simulink model "flightControlSystem"  (R2019a)
settings: Solver=ode3  StartTime=0  StopTime=TFinal  FixedStep=Ts  RelTol=1e-3  EnableMultiTasking=on
undefined symbols (not defined in the file): codertarget, Controller, DiscIntNeverNeededParam, Discrete, Estimator, g, init, Sensors, Time, Ts, Vehicle
libraries: simulink x37, sharedtransform x3, ctrlSharedLib x2, sharedutil x1, parrotlib x1
(part 1 of 2)
settings Model: ExtModeTrigDuration=80  Creator=The MathWorks, Inc.  LastModifiedBy=jeiso
settings SolverCC: AutoInsertRateTranBlk=on
settings DataIOCC: LimitDataPoints=on  SaveFormat=StructureWithTime  ReturnWorkspaceOutputs=off
settings OptimizationCC: BlockReduction=off  EnhancedBackFolding=on  PassReuseOutputArgsAs=Individual arguments  MaxStackSize=64  OptimizeBlockOrder=speed  DifferentSizesBufferReuse=on  OptimizationCustomize=off
settings DebuggingCC: AlgebraicLoopMsg=none  ParameterPrecisionLossMsg=none  ParameterTunabilityLossMsg=error  UnconnectedInputMsg=none  UnconnectedOutputMsg=none  UnconnectedLineMsg=none  BusObjectLabelMismatch=error  PregeneratedLibrarySubsystemCodeDiagnostic=none  SFUnexpectedBacktrackingDiag=warning  SFNoUnconditionalDefaultTransitionDiag=warning  SFExecutionAtInitializationDiag=none  ArithmeticOperatorsInVariantConditions=warning
settings HardwareCC: ProdBitPerPointer=32  ProdBitPerSizeT=32  ProdBitPerPtrDiffT=32  ProdLargestAtomicInteger=Long  ProdWordSize=32  ProdHWDeviceType=ARM Compatible->ARM 9  UseEmbeddedCoderFeatures=off  UseSimulinkCoderFeatures=off
settings ModelReferenceCC: ModelReferenceNumInstancesAllowed=Single  PropagateSignalLabelsOutOfModel=off
settings SFSimCC: SimUseLocalCustomCode=off  MATLABDynamicMemAlloc=off
settings RTWCC: SystemTargetFile=ert.tlc  HardwareBoard=PARROT Mambo  TLCOptions=-aInlineSetEventsForThisBaseRateFcn=TLC_FALSE -aSuppressMultiTaskScheduler=TLC_FALSE -aRateBasedStepFcn=1  TemplateMakefile=ert_default_tmf  RTWUseLocalCustomCode=off  Toolchain=Sourcery G++ Lite GNU Toolchain for Drones  IncludeHyperlinkInReport=on
settings CodeAppCC: ForceParamTrailComments=on  IgnoreCustomStorageClasses=off  MaxIdLength=63  OperatorAnnotations=on  SimulinkDataObjDesc=on  SFDataObjDesc=on  InsertBlockDesc=on
settings ERTTargetCC: MatFileLogging=on  SupportNonInlinedSFcns=on
settings ConfigComp: CovMetricSettings=dw  CovHtmlReporting=on  CovSaveCumulativeToWorkspaceVar=on  CovSaveSingleToWorkspaceVar=on  CovExternalEMLEnable=off  CovSFcnEnable=off

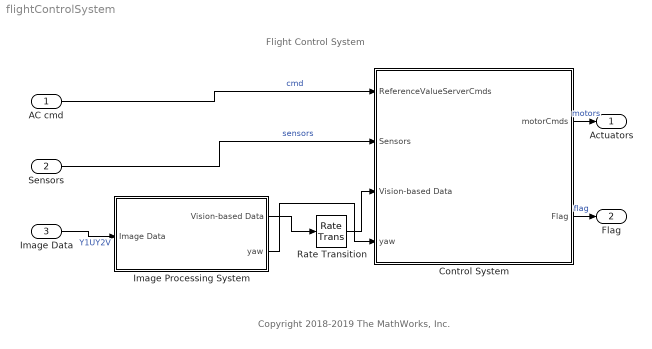
== system flightControlSystem ==
  note: Copyright 2018-2019 The MathWorks, Inc.
  note: Flight Control System
  AC cmd : Inport  OutDataTypeStr=Bus: CommandBus  BusOutputAsStruct=on
  Sensors : Inport  Port=2  OutDataTypeStr=Bus: SensorsBus  BusOutputAsStruct=on
  Image Data : Inport  Tag=IP_IN  InitFcn=codertarget.parrot.internal.inportCallback(gcb);  Port=3  OutDataTypeStr=uint8  PortDimensions=[4 9600]  BusOutputAsStruct=on
  Control System : Subsystem  InitFcn=codertarget.parrot.internal.fcsSubsystemCallback(gcb);  TreatAsAtomicUnit=on  SystemSampleTime=Ts
  Image Processing System : Subsystem  Tag=IP_SUB  InitFcn=codertarget.parrot.internal.ipSubsystemCallback(gcb);  TreatAsAtomicUnit=on  SystemSampleTime=40*Ts  RTWFcnName=ImageFunction
      settings: RTWSystemCode=Inline  RTWFcnNameOpts=User specified
  Rate Transition : RateTransition  Deterministic=off
  Actuators : Outport  OutDataTypeStr=single  PortDimensions=4
  Flag : Outport  Port=2  OutDataTypeStr=uint8  PortDimensions=1
  wires:
  AC cmd/1 -> Control System/1(ReferenceValueServerCmds)  "cmd"
  Control System/1(motorCmds) -> Actuators/1  "motors"
  Sensors/1 -> Control System/2(Sensors)  "sensors"
  Control System/2(Flag) -> Flag/1  "flag"
  Image Data/1 -> Image Processing System/1(Image Data)  "Y1UY2V"
  Image Processing System/1(Vision-based Data) -> Rate Transition/1
  Rate Transition/1 -> Control System/3(Vision-based Data)
  Image Processing System/2("yaw ") -> Control System/4(" yaw")

== system flightControlSystem/Control System ==
  note: Position or Orientation Control
  note: Use this subsystem to change the path of the
      | Minidrone depending on the input Vision-based
      | Data
  note: Derived from the work by Sertac
      | Karaman and Fabian Riether
  ReferenceValueServerCmds : Inport  OutDataTypeStr=Bus: CommandBus
  Sensors : Inport  Port=2  OutDataTypeStr=Bus: SensorsBus  BusOutputAsStruct=on
  Vision-based Data : Inport  Port=3
  " yaw" : Inport  Port=4
  Bus Selector1 : BusSelector  OutputSignals=opticalFlow_data
  Bus Selector4 : BusSelector  OutputSignals=VisionSensors,SensorCalibration
  Control Mode Update : BusAssignment  AssignedSignals=controlModePosVSOrient
  Controller : Subsystem
  Crash Predictor Flags : Subsystem
  Path Planning : Subsystem
  State Estimator : Subsystem
  To Workspace : ToWorkspace  VariableName=estimatedStates  SaveFormat=Structure With Time  SampleTime=-1
  controlModePosVsOrient : Constant  OutDataTypeStr=boolean
  motorCmds : Outport
  Flag : Outport  Port=2
  wires:
  ReferenceValueServerCmds/1 -> Control Mode Update/1
  Bus Selector1/1 -> State Estimator/3(opticalFlow_datin)  "<opticalFlow_data>"
  Bus Selector4/2 -> State Estimator/4(sensorCalibration_datin)  "<SensorCalibration>"
  Path Planning/1(UpdatedReferenceCmds) -> Controller/1(ReferenceValueServerBus)
  Bus Selector4/1 -> Bus Selector1/1  "<VisionSensors>"
  Vision-based Data/1 -> Path Planning/4(rojo)
  Crash Predictor Flags/1(Flag) -> Flag/1
  Control Mode Update/1 -> Path Planning/1(ReferenceValueServerCmds)
  controlModePosVsOrient/1 -> State Estimator/1(controlModePosVSOrient_flagin), Control Mode Update/2
  Controller/1(motors_refout) -> motorCmds/1
  Sensors/1 -> State Estimator/2(sensor_data_in), Crash Predictor Flags/3(Sensors), Bus Selector4/1
  State Estimator/1(states_estim) -> Path Planning/2(EstimatedVal), Controller/2(states_estim), Crash Predictor Flags/1(states_estim), To Workspace/1
  State Estimator/2(Alt_prs) -> Crash Predictor Flags/2(Alt_prs)
  " yaw"/1 -> Path Planning/3(grados)
  Path Planning/2("yaw ") -> Controller/3("yaw ")

== system flightControlSystem/Image Processing System ==
  note: Find the dominance of blue in the image
  note: Find the B-(R/2)-(G/2) image
  note: Obtain the RGB image from camera
  Image Data : Inport
  Add : Sum  Inputs=--+
  Constant : Constant  Value=2
  Delay : Delay  DelayLength=1
  Deteccion de giros : MATLAB Function  TreatAsAtomicUnit=on
  Display : Display
  Display1 : Display
  Divide1 : Product  Inputs=/*
  Divide2 : Product  Inputs=*/
  PARROT Image Conversion : parrotlib/PARROT Image Conversion  ImageFormat=RGB  R=on  Y=on  G=on  U=on  B=on  V=on
      settings: SourceProductName=Simulink Support Package for PARROT Minidrones
  RGB Image : VideoViewer  FigPos=[565 571 418 304]
  RGB Image1 : VideoViewer  FigPos=[896 489 418 304]
  Sum of white pixels : Sum  Inputs=+  OutDataTypeStr=uint16
  Threshold for each pixel : simulink/Logic and Bit Operations/Compare To Constant  relop=>  const=50  OutDataTypeStr=boolean
  Threshold for total white pixels : simulink/Logic and Bit Operations/Compare To Constant  relop=>  const=1400  OutDataTypeStr=boolean
  To Workspace : ToWorkspace  VariableName=simout  SaveFormat=Timeseries  SampleTime=-1
  Vision-based Data : Outport
  "yaw " : Outport  Port=2
  wires:
  Image Data/1 -> PARROT Image Conversion/1
  Threshold for total white pixels/1 -> Vision-based Data/1
  Add/1 -> Threshold for each pixel/1
  Sum of white pixels/1 -> Threshold for total white pixels/1
  Divide2/1 -> Add/1
  PARROT Image Conversion/3 -> Divide2/1
  PARROT Image Conversion/1 -> Add/3
  PARROT Image Conversion/2 -> Divide1/2
  Divide1/1 -> Add/2
  Constant/1 -> Divide1/1, Divide2/2
  Deteccion de giros/2(grados) -> Delay/1, "yaw "/1
  Deteccion de giros/4(imagen) -> RGB Image1/1
  Threshold for each pixel/1 -> Deteccion de giros/1(img), RGB Image/1, Sum of white pixels/1
  Deteccion de giros/3(lado) -> Display1/1
  Delay/1 -> Deteccion de giros/2(grado)
  Deteccion de giros/1(ade) -> To Workspace/1, Display/1

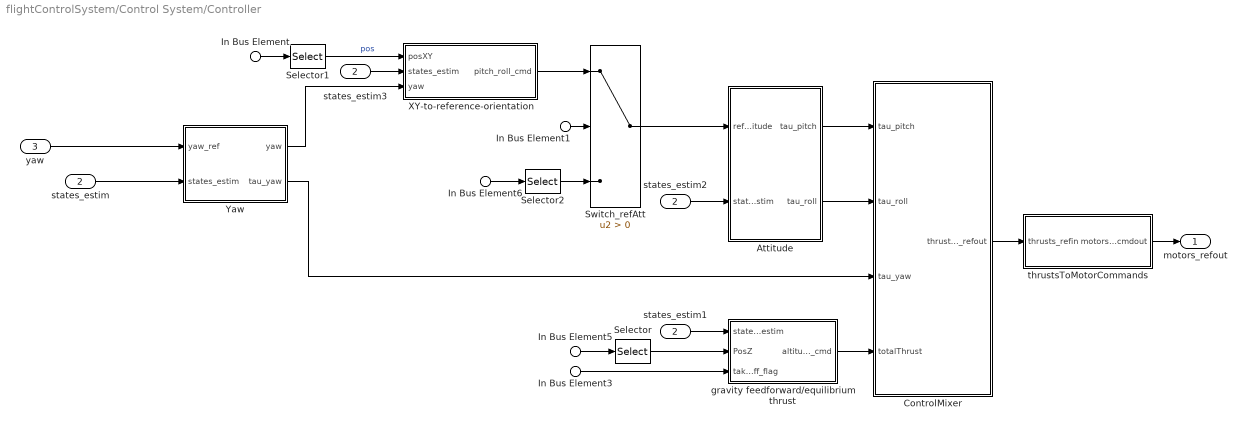
== system flightControlSystem/Control System/Controller ==
  In Bus Element1 : Inport  PortName=ReferenceValueServerBus  Element=controlModePosVSOrient
  In Bus Element : Inport  PortName=ReferenceValueServerBus  Element=pos_ref
  In Bus Element5 : Inport  PortName=ReferenceValueServerBus  Element=pos_ref
  In Bus Element6 : Inport  PortName=ReferenceValueServerBus  Element=orient_ref
  In Bus Element3 : Inport  PortName=ReferenceValueServerBus  Element=takeoff_flag
  states_estim : Inport  Port=2
  "yaw " : Inport  Port=3
  Attitude : Subsystem
  ControlMixer : Subsystem
  Selector : Selector  InputPortWidth=3  IndexOptions=Index vector (dialog)  Indices=3  OutputSizes=1
  Selector1 : Selector  InputPortWidth=3  IndexOptions=Index vector (dialog)  Indices=[1 2]  OutputSizes=1
  Selector2 : Selector  InputPortWidth=3  IndexOptions=Index vector (dialog)  Indices=[2 3]  OutputSizes=1
  Switch_refAtt : Switch  Criteria=u2 > Threshold
  XY-to-reference-orientation : Subsystem
  Yaw : Subsystem
  gravity feedforward/equilibrium thrust : Subsystem
  states_estim1 : InportShadow  Port=2
  states_estim2 : InportShadow  Port=2
  states_estim3 : InportShadow  Port=2
  thrustsToMotorCommands : Subsystem
  motors_refout : Outport
  wires:
  thrustsToMotorCommands/1(motors_cmdout) -> motors_refout/1
  In Bus Element5/1 -> Selector/1
  Attitude/2(tau_roll) -> ControlMixer/2(tau_roll)
  states_estim3/1 -> XY-to-reference-orientation/2(states_estim)
  In Bus Element6/1 -> Selector2/1
  "yaw "/1 -> Yaw/1(yaw_ref)
  In Bus Element/1 -> Selector1/1
  ControlMixer/1(thrusts_refout) -> thrustsToMotorCommands/1(thrusts_refin)
  Selector2/1 -> Switch_refAtt/3
  Attitude/1(tau_pitch) -> ControlMixer/1(tau_pitch)
  gravity feedforward/equilibrium thrust/1(altitude_cmd) -> ControlMixer/4(totalThrust)
  Selector1/1 -> XY-to-reference-orientation/1(posXY)  "pos"
  states_estim1/1 -> gravity feedforward/equilibrium thrust/1(states_estim)
  Selector/1 -> gravity feedforward/equilibrium thrust/2(PosZ)
  Yaw/1(yaw) -> XY-to-reference-orientation/3(yaw)
  In Bus Element3/1 -> gravity feedforward/equilibrium thrust/3(takeoff_flag)
  states_estim/1 -> Yaw/2(states_estim)
  XY-to-reference-orientation/1(pitch_roll_cmd) -> Switch_refAtt/1
  Yaw/2(tau_yaw) -> ControlMixer/3(tau_yaw)
  In Bus Element1/1 -> Switch_refAtt/2
  Switch_refAtt/1 -> Attitude/1(refAttitude)
  states_estim2/1 -> Attitude/2(states_estim)

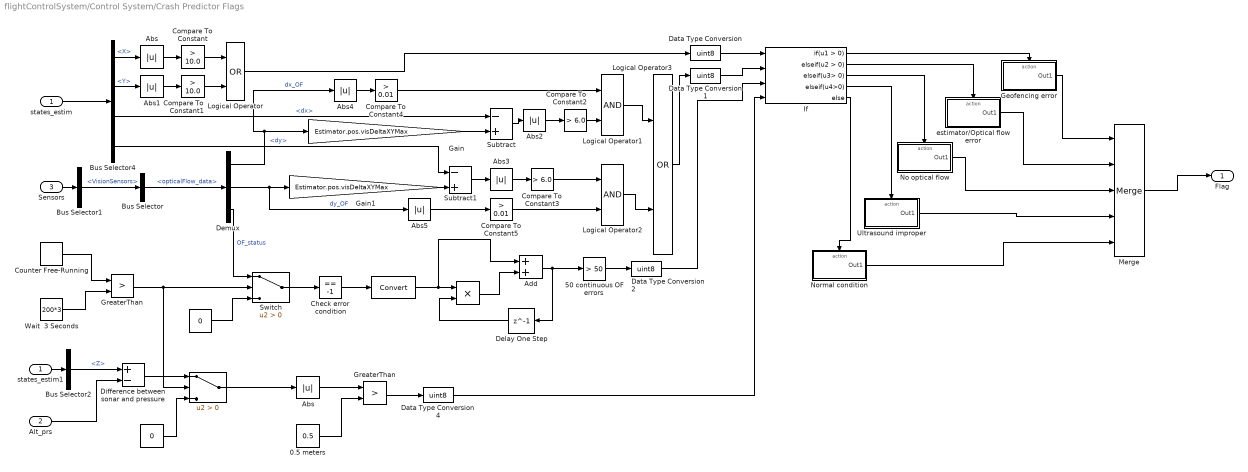
== system flightControlSystem/Control System/Crash Predictor Flags ==
  states_estim : Inport
  Alt_prs : Inport  Port=2
  Sensors : Inport  Port=3
  " " : Constant  Value=0
  "  " : Product  Inputs=**
  "   " : DataTypeConversion
  "    " : Constant  Value=0  OutDataTypeStr=single
  "         " : Switch  Criteria=u2 > Threshold
  0.5 meters : Constant  Value=0.5
  "50 continuous OF errors " : simulink/Logic and Bit Operations/Compare To Constant  relop=>  const=50  OutDataTypeStr=boolean
  Abs{,1..5} (6 alike) : Abs
  "Abs  " : Abs
  Add : Sum
  Bus Selector : BusSelector  OutputSignals=opticalFlow_data
  Bus Selector1 : BusSelector  OutputSignals=VisionSensors
  Bus Selector2 : BusSelector  OutputSignals=Z
  Bus Selector4 : BusSelector  OutputSignals=X,Y,dx,dy
  Check error condition : simulink/Logic and Bit Operations/Compare To Constant  relop===  const=-1  OutDataTypeStr=boolean
  Compare To Constant : simulink/Logic and Bit Operations/Compare To Constant  relop=>  const=10.0  OutDataTypeStr=boolean
  Compare To Constant1 : simulink/Logic and Bit Operations/Compare To Constant  relop=>  const=10.0  OutDataTypeStr=boolean
  Compare To Constant2 : simulink/Logic and Bit Operations/Compare To Constant  relop=>  const=6.0  OutDataTypeStr=boolean
  Compare To Constant3 : simulink/Logic and Bit Operations/Compare To Constant  relop=>  const=6.0  OutDataTypeStr=boolean
  Compare To Constant4 : simulink/Logic and Bit Operations/Compare To Constant  relop=>  const=0.01  OutDataTypeStr=boolean
  Compare To Constant5 : simulink/Logic and Bit Operations/Compare To Constant  relop=>  const=0.01  OutDataTypeStr=boolean
  Counter Free-Running : simulink/Sources/Counter Free-Running  NumBits=32  tsamp=-1
  Data Type Conversion{,1..2,4} (4 alike) : DataTypeConversion  OutDataTypeStr=uint8  RndMeth=Nearest
  Delay One Step : Delay  DelayLength=1
  Demux : Demux  Outputs=3
  Difference between sonar and pressure : Sum  Inputs=+-
  Gain : Gain  Gain=Estimator.pos.visDeltaXYMax
  Gain1 : Gain  Gain=Estimator.pos.visDeltaXYMax
  Geofencing error : Subsystem  TreatAsAtomicUnit=on
  GreaterThan : RelationalOperator  Operator=>  OutDataTypeStr=boolean  RndMeth=Simplest
  "GreaterThan  " : RelationalOperator  Operator=>  OutDataTypeStr=boolean  RndMeth=Simplest
  If : If  NumInputs=4  ElseIfExpressions=u2 > 0, u3> 0,u4>0
  Logical Operator : Logic  Operator=OR  AllPortsSameDT=off
  Logical Operator1 : Logic  AllPortsSameDT=off  OutDataTypeStr=boolean
  Logical Operator2 : Logic  AllPortsSameDT=off  OutDataTypeStr=boolean
  Logical Operator3 : Logic  Operator=OR  AllPortsSameDT=off
  Merge : Merge  Inputs=5  InitialOutput=0
  "No optical flow " : Subsystem  TreatAsAtomicUnit=on
  Normal condition : Subsystem  TreatAsAtomicUnit=on
  Subtract : Sum  Inputs=-+
  Subtract1 : Sum  Inputs=-+
  Switch : Switch  Criteria=u2 > Threshold
  Ultrasound improper : Subsystem  TreatAsAtomicUnit=on
  Wait  3 Seconds : Constant  Value=200*3
  estimator/Optical flow error : Subsystem  TreatAsAtomicUnit=on
  states_estim1 : InportShadow
  Flag : Outport
  wires:
  Bus Selector4/1 -> Abs/1  "<X>"
  states_estim/1 -> Bus Selector4/1
  Bus Selector4/2 -> Abs1/1  "<Y>"
  Compare To Constant/1 -> Logical Operator/1
  Compare To Constant1/1 -> Logical Operator/2
  Abs/1 -> Compare To Constant/1
  Abs1/1 -> Compare To Constant1/1
  Logical Operator/1 -> Data Type Conversion/1
  Bus Selector/1 -> Demux/1  "<opticalFlow_data>"
  Demux/1 -> Abs4/1, Gain/1  "dx_OF"
  Demux/2 -> Gain1/1, Abs5/1  "dy_OF"
  Bus Selector4/3 -> Subtract/1  "<dx>"
  Subtract/1 -> Abs2/1
  Subtract1/1 -> Abs3/1
  Abs2/1 -> Compare To Constant2/1
  Abs3/1 -> Compare To Constant3/1
  Compare To Constant5/1 -> Logical Operator2/2
  Abs4/1 -> Compare To Constant4/1
  Abs5/1 -> Compare To Constant5/1
  Compare To Constant3/1 -> Logical Operator2/1
  Logical Operator1/1 -> Logical Operator3/1
  Logical Operator2/1 -> Logical Operator3/2
  Logical Operator3/1 -> Data Type Conversion1/1
  Gain/1 -> Subtract/2
  Bus Selector4/4 -> Subtract1/1  "<dy>"
  Gain1/1 -> Subtract1/2
  Compare To Constant4/1 -> Logical Operator1/1
  Compare To Constant2/1 -> Logical Operator1/2
  Sensors/1 -> Bus Selector1/1
  Bus Selector1/1 -> Bus Selector/1  "<VisionSensors>"
  Merge/1 -> Flag/1
  If/1 -> Geofencing error/Action
  If/2 -> estimator/Optical flow error/Action
  If/5 -> Normal condition/Action
  Geofencing error/1(Out1) -> Merge/1
  estimator/Optical flow error/1(Out1) -> Merge/2
  Normal condition/1(Out1) -> Merge/5
  Data Type Conversion/1 -> If/1
  Data Type Conversion1/1 -> If/2
  Check error condition/1 -> "   "/1
  Demux/3 -> Switch/1  "OF_status"
  Delay One Step/1 -> "  "/2
  Add/1 -> Delay One Step/1, "50 continuous OF errors "/1
  "  "/1 -> Add/2
  "50 continuous OF errors "/1 -> Data Type Conversion2/1
  Data Type Conversion2/1 -> If/3
  "No optical flow "/1(Out1) -> Merge/3
  If/3 -> "No optical flow "/Action
  "   "/1 -> Add/1, "  "/1
  Counter Free-Running/1 -> GreaterThan/1
  Wait  3 Seconds/1 -> GreaterThan/2
  Switch/1 -> Check error condition/1
  " "/1 -> Switch/3
  "    "/1 -> "         "/3
  Difference between sonar and pressure/1 -> "         "/1
  Bus Selector2/1 -> Difference between sonar and pressure/1  "<Z>"
  GreaterThan/1 -> Switch/2, "         "/2
  "         "/1 -> "Abs  "/1
  "Abs  "/1 -> "GreaterThan  "/1
  0.5 meters/1 -> "GreaterThan  "/2
  Alt_prs/1 -> Difference between sonar and pressure/2
  "GreaterThan  "/1 -> Data Type Conversion4/1
  states_estim1/1 -> Bus Selector2/1
  Data Type Conversion4/1 -> If/4
  Ultrasound improper/1(Out1) -> Merge/4
  If/4 -> Ultrasound improper/Action

== system flightControlSystem/Control System/Path Planning ==
  note: Estimated values from the
      | State Estimator
  ReferenceValueServerCmds : Inport
  EstimatedVal : Inport  Port=2
  grados : Inport  Port=3
  rojo : Inport  Port=4
  Bus Selector1 : BusSelector  OutputSignals=X,Y,Z,yaw,pitch,roll
  Bus Assignment : BusAssignment  AssignedSignals=pos_ref
  Chart : Stateflow chart  BlockKeywords=__PRM__SERIALIZED__DATA__:Stateflow Chart,Stateflow Diagram  TreatAsAtomicUnit=on
  Mux : Mux  Inputs=3
  Terminator3 : Terminator
  Terminator5 : Terminator
  Terminator6 : Terminator
  UpdatedReferenceCmds : Outport
  "yaw " : Outport  Port=2
  wires:
  Bus Assignment/1 -> UpdatedReferenceCmds/1
  ReferenceValueServerCmds/1 -> Bus Assignment/1
  EstimatedVal/1 -> Bus Selector1/1
  Bus Selector1/1 -> Chart/1(xest)  "<X>"
  Bus Selector1/2 -> Chart/2(yest)  "<Y>"
  Bus Selector1/3 -> Terminator3/1  "<Z>"
  Bus Selector1/4 -> Chart/5(yawest)  "<yaw>"
  Bus Selector1/5 -> Terminator5/1  "<pitch>"
  Bus Selector1/6 -> Terminator6/1  "<roll>"
  Mux/1 -> Bus Assignment/2
  grados/1 -> Chart/4(grados)
  Chart/4(yaw) -> "yaw "/1
  Chart/1(x) -> Mux/1
  Chart/2(y) -> Mux/2
  Chart/3(z) -> Mux/3
  rojo/1 -> Chart/3(rojo)

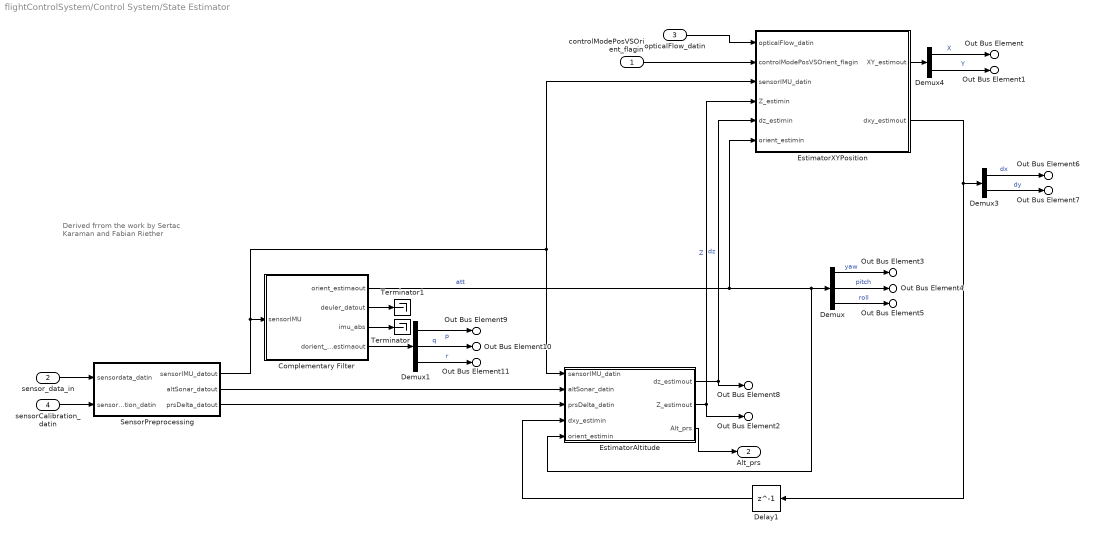
== system flightControlSystem/Control System/State Estimator ==
  note: Derived frrom the work by Sertac
      | Karaman and Fabian Riether
  controlModePosVSOrient_flagin : Inport  OutDataTypeStr=boolean
  sensor_data_in : Inport  Port=2
  opticalFlow_datin : Inport  Port=3
  sensorCalibration_datin : Inport  Port=4
  Complementary Filter : Subsystem
  Delay1 : Delay  DelayLength=1  InitialCondition=0
  Demux : Demux  Outputs=3
  Demux1 : Demux  Outputs=3
  Demux3 : Demux  Outputs=2
  Demux4 : Demux  Outputs=2
  EstimatorAltitude : Subsystem
  EstimatorXYPosition : Subsystem
  SensorPreprocessing : Subsystem
  Terminator : Terminator
  Terminator1 : Terminator
  Out Bus Element : Outport  PortName=states_estim  Element=X
  Out Bus Element1 : Outport  PortName=states_estim  Element=Y
  Out Bus Element2 : Outport  PortName=states_estim  Element=Z
  Out Bus Element3 : Outport  PortName=states_estim  Element=yaw
  Out Bus Element4 : Outport  PortName=states_estim  Element=pitch
  Out Bus Element5 : Outport  PortName=states_estim  Element=roll
  Out Bus Element6 : Outport  PortName=states_estim  Element=dx
  Out Bus Element7 : Outport  PortName=states_estim  Element=dy
  Out Bus Element8 : Outport  PortName=states_estim  Element=dz
  Out Bus Element9 : Outport  PortName=states_estim  Element=p
  Out Bus Element10 : Outport  PortName=states_estim  Element=q
  Out Bus Element11 : Outport  PortName=states_estim  Element=r
  Alt_prs : Outport  Port=2
  wires:
  EstimatorXYPosition/2(dxy_estimout) -> Delay1/1, Demux3/1
  Demux1/3 -> Out Bus Element11/1  "r"
  Demux/3 -> Out Bus Element5/1  "roll"
  Demux4/2 -> Out Bus Element1/1  "Y"
  EstimatorXYPosition/1(XY_estimout) -> Demux4/1
  Complementary Filter/2(deuler_datout) -> Terminator1/1
  Complementary Filter/4(dorient_estimaout) -> Demux1/1
  sensor_data_in/1 -> SensorPreprocessing/1(sensordata_datin)
  opticalFlow_datin/1 -> EstimatorXYPosition/1(opticalFlow_datin)
  Demux4/1 -> Out Bus Element/1  "X"
  SensorPreprocessing/1(sensorIMU_datout) -> EstimatorAltitude/1(sensorIMU_datin), EstimatorXYPosition/3(sensorIMU_datin), Complementary Filter/1(sensorIMU)
  SensorPreprocessing/3(prsDelta_datout) -> EstimatorAltitude/3(prsDelta_datin)
  Demux3/2 -> Out Bus Element7/1  "dy"
  SensorPreprocessing/2(altSonar_datout) -> EstimatorAltitude/2(altSonar_datin)
  EstimatorAltitude/1(dz_estimout) -> EstimatorXYPosition/5(dz_estimin), Out Bus Element8/1  "dz"
  EstimatorAltitude/2(Z_estimout) -> Out Bus Element2/1, EstimatorXYPosition/4(Z_estimin)  "Z"
  Demux1/1 -> Out Bus Element9/1  "p"
  Demux3/1 -> Out Bus Element6/1  "dx"
  Complementary Filter/3(imu_abs) -> Terminator/1
  Demux/2 -> Out Bus Element4/1  "pitch"
  controlModePosVSOrient_flagin/1 -> EstimatorXYPosition/2(controlModePosVSOrient_flagin)
  Complementary Filter/1(orient_estimaout) -> EstimatorAltitude/5(orient_estimin), Demux/1, EstimatorXYPosition/6(orient_estimin)  "att"
  Demux/1 -> Out Bus Element3/1  "yaw"
  Delay1/1 -> EstimatorAltitude/4(dxy_estimin)
  Demux1/2 -> Out Bus Element10/1  "q"
  sensorCalibration_datin/1 -> SensorPreprocessing/2(sensorCalibration_datin)
  EstimatorAltitude/3(Alt_prs) -> Alt_prs/1

== system flightControlSystem/Control System/Controller/Attitude ==
  note: ATTITUDE
  refAttitude : Inport
  states_estim : Inport  Port=2
  Add : Sum  Inputs=+-
  Bus Selector3 : BusSelector  OutputSignals=pitch,roll
  Bus Selector4 : BusSelector  OutputSignals=q,p
  D_pr : Gain  Gain=[0.002;0.003]
  Delay : Delay  DelayLength=1  InitialCondition=0
  Demux : Demux  Outputs=2
  Discrete-Time Integrator : DiscreteIntegrator  SampleTime=Ts  LimitOutput=on  UpperSaturationLimit=2  LowerSaturationLimit=-2  ICPrevOutput=DiscIntNeverNeededParam  ICPrevScaledInput=DiscIntNeverNeededParam
  I_pr : Gain  Gain=0.01
  Mux : Mux  Inputs=2
  Mux1 : Mux  Inputs=2
  P_pr : Gain  Gain=[0.013;0.011]
  Sum16 : Sum  Inputs=++-  AccumDataTypeStr=single  OutDataTypeStr=single  SaturateOnIntegerOverflow=on
  Sum19 : Sum  Inputs=+-|
  antiWU_Gain : Gain  Gain=0.001
  tau_pitch : Outport
  tau_roll : Outport  Port=2
  wires:
  Sum16/1 -> Demux/1  "P_pr"
  antiWU_Gain/1 -> Add/2
  Add/1 -> Discrete-Time Integrator/1
  Bus Selector3/1 -> Mux/1  "<pitch>"
  Bus Selector4/1 -> Mux1/1  "<q>"
  P_pr/1 -> Sum16/1
  I_pr/1 -> Sum16/2
  Sum19/1 -> Add/1, P_pr/1  "pitch/roll error"
  Discrete-Time Integrator/1 -> Delay/1, I_pr/1
  Delay/1 -> antiWU_Gain/1
  Demux/1 -> tau_pitch/1  "tau_pitch"
  Demux/2 -> tau_roll/1
  D_pr/1 -> Sum16/3
  states_estim/1 -> Bus Selector3/1, Bus Selector4/1
  refAttitude/1 -> Sum19/1
  Mux/1 -> Sum19/2
  Bus Selector3/2 -> Mux/2  "<roll>"
  Mux1/1 -> D_pr/1
  Bus Selector4/2 -> Mux1/2  "<p>"

== system flightControlSystem/Control System/Controller/ControlMixer ==
  tau_pitch : Inport
  tau_roll : Inport  Port=2
  tau_yaw : Inport  Port=3
  totalThrust : Inport  Port=4
  Mux2 : Mux
  Product : Product  Multiplication=Matrix(*)  RndMeth=Zero
  TorqueTotalThrustToThrustPerMotor : Constant  Value=Controller.Q2Ts  OutDataTypeStr=single
  thrusts_refout : Outport
  wires:
  Product/1 -> thrusts_refout/1
  tau_roll/1 -> Mux2/4
  tau_pitch/1 -> Mux2/3
  tau_yaw/1 -> Mux2/2
  totalThrust/1 -> Mux2/1
  TorqueTotalThrustToThrustPerMotor/1 -> Product/1
  Mux2/1 -> Product/2

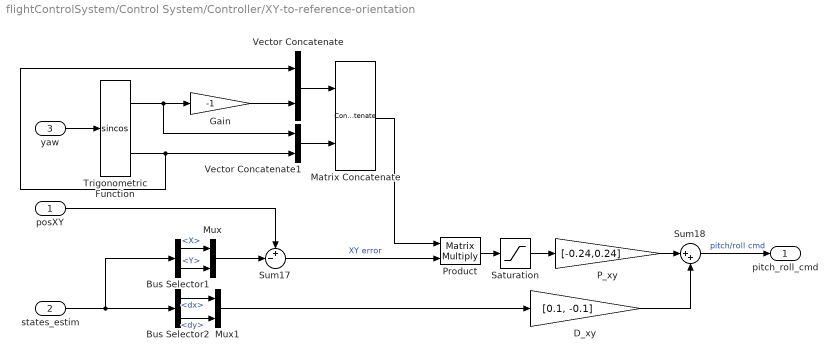
== system flightControlSystem/Control System/Controller/XY-to-reference-orientation ==
  posXY : Inport
  states_estim : Inport  Port=2
  yaw : Inport  Port=3
  Bus Selector1 : BusSelector  OutputSignals=X,Y
  Bus Selector2 : BusSelector  OutputSignals=dx,dy
  D_xy : Gain  Gain=[0.1, -0.1]  ParamDataTypeStr=single  OutDataTypeStr=single  SaturateOnIntegerOverflow=on
  Gain : Gain  Gain=-1
  Matrix Concatenate : Concatenate  Mode=Multidimensional array  ConcatenateDimension=2
  Mux : Mux  Inputs=2
  Mux1 : Mux  Inputs=2
  P_xy : Gain  Gain=[-0.24,0.24]  ParamDataTypeStr=single  OutDataTypeStr=single  SaturateOnIntegerOverflow=on
  Product : Product  Multiplication=Matrix(*)  OutDataTypeStr=single  RndMeth=Zero
  Saturation : Saturate  UpperLimit=3  LowerLimit=-3  OutDataTypeStr=single
  Sum17 : Sum  Inputs=+-|  AccumDataTypeStr=single
  Sum18 : Sum  Inputs=|++  AccumDataTypeStr=single  OutDataTypeStr=single  SaturateOnIntegerOverflow=on
  Trigonometric Function : Trigonometry  Operator=sincos
  Vector Concatenate : Concatenate
  Vector Concatenate1 : Concatenate
  pitch_roll_cmd : Outport
  wires:
  yaw/1 -> Trigonometric Function/1
  Saturation/1 -> P_xy/1
  P_xy/1 -> Sum18/1
  Sum17/1 -> Product/2  "XY error"
  posXY/1 -> Sum17/1
  Bus Selector2/1 -> Mux1/1  "<dx>"
  states_estim/1 -> Bus Selector1/1, Bus Selector2/1
  Sum18/1 -> pitch_roll_cmd/1  "pitch/roll cmd"
  D_xy/1 -> Sum18/2
  Bus Selector1/1 -> Mux/1  "<X>"
  Product/1 -> Saturation/1
  Trigonometric Function/1 -> Gain/1, Vector Concatenate1/1
  Trigonometric Function/2 -> Vector Concatenate1/2, Vector Concatenate/1
  Gain/1 -> Vector Concatenate/2
  Vector Concatenate/1 -> Matrix Concatenate/1
  Vector Concatenate1/1 -> Matrix Concatenate/2
  Matrix Concatenate/1 -> Product/1
  Bus Selector1/2 -> Mux/2  "<Y>"
  Mux/1 -> Sum17/2
  Mux1/1 -> D_xy/1
  Bus Selector2/2 -> Mux1/2  "<dy>"

== system flightControlSystem/Control System/Controller/Yaw ==
  yaw_ref : Inport
  states_estim : Inport  Port=2
  Bus Selector5 : BusSelector  OutputSignals=yaw,r
  D_yaw : Gain  Gain=0.3*0.004
  P_yaw : Gain  Gain=0.004  ParamDataTypeStr=single  OutDataTypeStr=single
  Sum1 : Sum  Inputs=+-|  AccumDataTypeStr=single  OutDataTypeStr=single  SaturateOnIntegerOverflow=on
  Sum2 : Sum  Inputs=|+-
  yaw : Outport
  tau_yaw : Outport  Port=2
  wires:
  D_yaw/1 -> Sum2/2
  P_yaw/1 -> Sum2/1
  Bus Selector5/2 -> D_yaw/1  "<r>"
  Sum1/1 -> P_yaw/1
  states_estim/1 -> Bus Selector5/1
  Sum2/1 -> tau_yaw/1
  Bus Selector5/1 -> yaw/1, Sum1/2  "<yaw>"
  yaw_ref/1 -> Sum1/1

== system flightControlSystem/Control System/Controller/gravity feedforward//equilibrium thrust ==
  note: ALTITUDE
  states_estim : Inport
  PosZ : Inport  Port=2
  takeoff_flag : Inport  Port=3
  Bus Selector1 : BusSelector  OutputSignals=Z,dz
  Compare To Constant : simulink/Logic and Bit Operations/Compare To Constant  relop=<  const=100  OutDataTypeStr=boolean
  Counter Free-Running : simulink/Sources/Counter Free-Running  NumBits=32  tsamp=-1
  D_z1 : Gain  Gain=0.5  ParamDataTypeStr=single  OutDataTypeStr=single  SaturateOnIntegerOverflow=on
  Discrete-Time Integrator : DiscreteIntegrator  ExternalReset=falling  SampleTime=Ts  LimitOutput=on  UpperSaturationLimit=2  LowerSaturationLimit=-2  ICPrevOutput=DiscIntNeverNeededParam  ICPrevScaledInput=DiscIntNeverNeededParam
  I_pr : Gain  Gain=0.24
  P_z1 : Gain  Gain=0.8  ParamDataTypeStr=single  OutDataTypeStr=single  SaturateOnIntegerOverflow=on
  SaturationThrust1 : Saturate  UpperLimit=4*Controller.totalThrustMaxRelative*Controller.motorsThrustPerMotorMax  LowerLimit=-4*Controller.totalThrustMaxRelative*Controller.motorsThrustPerMotorMax  OutDataTypeStr=single
  Sum1 : Sum  Inputs=++-  AccumDataTypeStr=single  OutDataTypeStr=single  SaturateOnIntegerOverflow=on
  Sum2 : Sum  Inputs=+-|  AccumDataTypeStr=single  OutDataTypeStr=single  SaturateOnIntegerOverflow=on
  Sum5 : Sum  Inputs=++|  AccumDataTypeStr=single  OutDataTypeStr=single  SaturateOnIntegerOverflow=on
  TakeoffOrControl_Switch1 : Switch  Criteria=u2 > Threshold
  Terminator : Terminator
  takeoff_gain1 : Gain  Gain=Controller.takeoffGain  ParamDataTypeStr=single  OutDataTypeStr=single  SaturateOnIntegerOverflow=on
  w1 : Constant  Value=-g*Vehicle.Airframe.mass  OutDataTypeStr=single  SampleTime=Ts
  altitude_cmd : Outport
  wires:
  I_pr/1 -> Discrete-Time Integrator/1
  Sum5/1 -> SaturationThrust1/1
  Compare To Constant/1 -> Discrete-Time Integrator/2, TakeoffOrControl_Switch1/2
  Discrete-Time Integrator/1 -> Sum1/1
  D_z1/1 -> Sum1/3  "dz"
  Sum2/1 -> I_pr/1, P_z1/1  "pitch/roll error"
  Bus Selector1/2 -> D_z1/1  "<dz>"
  takeoff_gain1/1 -> TakeoffOrControl_Switch1/1
  Sum1/1 -> TakeoffOrControl_Switch1/3
  Counter Free-Running/1 -> Compare To Constant/1
  P_z1/1 -> Sum1/2
  states_estim/1 -> Bus Selector1/1
  Bus Selector1/1 -> Sum2/2  "<Z>"
  PosZ/1 -> Sum2/1
  w1/1 -> Sum5/1, takeoff_gain1/1
  TakeoffOrControl_Switch1/1 -> Sum5/2
  SaturationThrust1/1 -> altitude_cmd/1
  takeoff_flag/1 -> Terminator/1

== system flightControlSystem/Control System/Controller/thrustsToMotorCommands ==
  thrusts_refin : Inport
  MotorDirections : Gain  Gain=[1 -1 1 -1]
  Saturation5 : Saturate  UpperLimit=Vehicle.Motor.maxLimit  LowerLimit=Vehicle.Motor.minLimit
  ThrustToMotorCommand : Gain  Gain=-Vehicle.Motor.thrustToMotorCommand
  motors_cmdout : Outport
  wires:
  Saturation5/1 -> MotorDirections/1
  MotorDirections/1 -> motors_cmdout/1
  ThrustToMotorCommand/1 -> Saturation5/1
  thrusts_refin/1 -> ThrustToMotorCommand/1

== system flightControlSystem/Control System/Crash Predictor Flags/Geofencing error ==
  Action Port : ActionPort  ActionPortLabel=if(u1 > 0)
  Constant : Constant  OutDataTypeStr=uint8
  Out1 : Outport
  wires:
  Constant/1 -> Out1/1

== system flightControlSystem/Control System/Crash Predictor Flags/No optical flow  ==
  Action Port : ActionPort  ActionPortLabel=elseif( u3> 0)
  Constant : Constant  Value=69  OutDataTypeStr=uint8
  Out1 : Outport
  wires:
  Constant/1 -> Out1/1

== system flightControlSystem/Control System/Crash Predictor Flags/Normal condition ==
  Action Port : ActionPort  ActionPortLabel=else
  Constant : Constant  Value=0  OutDataTypeStr=uint8
  Out1 : Outport
  wires:
  Constant/1 -> Out1/1

== system flightControlSystem/Control System/Crash Predictor Flags/Ultrasound improper ==
  Action Port : ActionPort  ActionPortLabel=elseif(u4>0)
  Constant : Constant  Value=88  OutDataTypeStr=uint8
  Out1 : Outport
  wires:
  Constant/1 -> Out1/1

== system flightControlSystem/Control System/Crash Predictor Flags/estimator//Optical flow error ==
  Action Port : ActionPort  ActionPortLabel=elseif(u2 > 0)
  Constant : Constant  Value=99  OutDataTypeStr=uint8
  Out1 : Outport
  wires:
  Constant/1 -> Out1/1

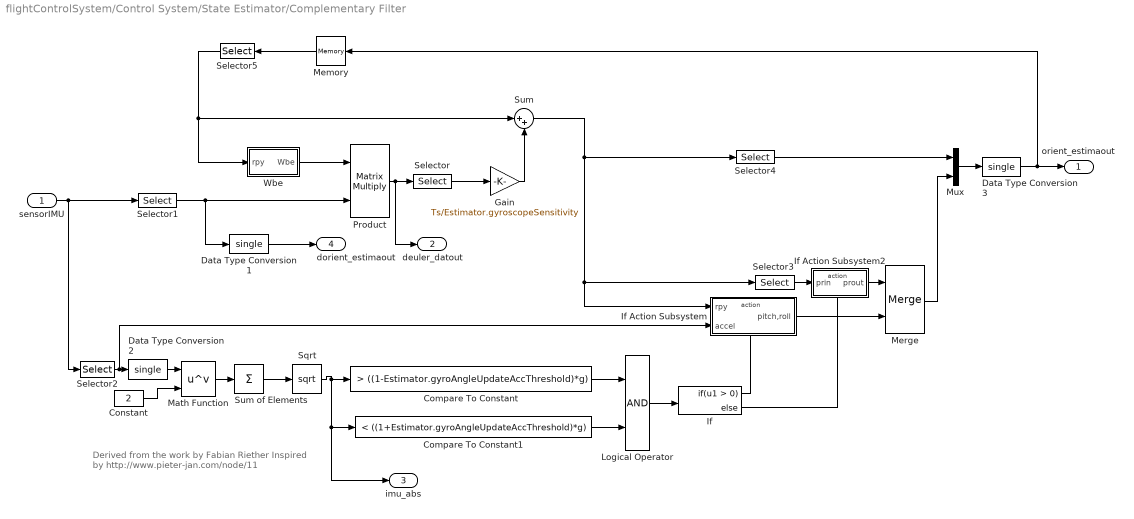
== system flightControlSystem/Control System/State Estimator/Complementary Filter ==
  note: Derived from the work by Fabian Riether
      | Inspired by http://www.pieter-jan.com/node/11
  sensorIMU : Inport  OutDataTypeStr=single
  Compare To Constant : simulink/Logic and Bit Operations/Compare To Constant  relop=>  const=((1-Estimator.gyroAngleUpdateAccThreshold)*g)  OutDataTypeStr=boolean
  Compare To Constant1 : simulink/Logic and Bit Operations/Compare To Constant  relop=<  const=((1+Estimator.gyroAngleUpdateAccThreshold)*g)  OutDataTypeStr=boolean
  Constant : Constant  Value=2  OutDataTypeStr=single
  Data Type Conversion1 : DataTypeConversion  OutDataTypeStr=single
  Data Type Conversion2 : DataTypeConversion  OutDataTypeStr=single
  Data Type Conversion3 : DataTypeConversion  OutDataTypeStr=single
  Gain : Gain  Gain=Ts/Estimator.gyroscopeSensitivity
  If : If
  If Action Subsystem : Subsystem  TreatAsAtomicUnit=on
  If Action Subsystem2 : Subsystem  TreatAsAtomicUnit=on
  Logical Operator : Logic  AllPortsSameDT=off  OutDataTypeStr=fixdt(1,16)
  Math Function : Math  Operator=pow  SaturateOnIntegerOverflow=on
  Memory : Memory  InitialCondition=single(Estimator.complementaryFilterInit)  InheritSampleTime=on
  Merge : Merge
  Mux : Mux  Inputs=2
  Product : Product  Multiplication=Matrix(*)
  Selector : Selector  InputPortWidth=3  IndexOptions=Index vector (dialog)  Indices=[3 2 1]  OutputSizes=1
  Selector1 : Selector  InputPortWidth=6  IndexOptions=Index vector (dialog)  Indices=[4 5 6]  OutputSizes=1
  Selector2 : Selector  InputPortWidth=6  IndexOptions=Index vector (dialog)  Indices=[1 2 3]  OutputSizes=1
  Selector3 : Selector  InputPortWidth=3  IndexOptions=Index vector (dialog)  Indices=[2 1]  OutputSizes=1
  Selector4 : Selector  InputPortWidth=3  IndexOptions=Index vector (dialog)  Indices=[3]  OutputSizes=1
  Selector5 : Selector  InputPortWidth=3  IndexOptions=Index vector (dialog)  Indices=[3 2 1]  OutputSizes=1
  Sqrt : Sqrt  SaturateOnIntegerOverflow=on
  Sum : Sum  Inputs=|++
  Sum of Elements : Sum  Inputs=+
  Wbe : Subsystem
  orient_estimaout : Outport
  deuler_datout : Outport  Port=2
  imu_abs : Outport  Port=3  OutDataTypeStr=single
  dorient_estimaout : Outport  Port=4
  wires:
  sensorIMU/1 -> Selector1/1, Selector2/1
  Product/1 -> deuler_datout/1, Selector/1
  Wbe/1(Wbe) -> Product/1
  Selector/1 -> Gain/1
  Gain/1 -> Sum/2
  Memory/1 -> Selector5/1
  Sum of Elements/1 -> Sqrt/1
  Math Function/1 -> Sum of Elements/1
  Constant/1 -> Math Function/2
  Selector2/1 -> If Action Subsystem/2(accel), Data Type Conversion2/1
  Sqrt/1 -> imu_abs/1, Compare To Constant1/1, Compare To Constant/1
  Compare To Constant/1 -> Logical Operator/1
  Compare To Constant1/1 -> Logical Operator/2
  If Action Subsystem/1(pitch,roll) -> Merge/2
  Sum/1 -> If Action Subsystem/1(rpy), Selector3/1, Selector4/1
  Selector3/1 -> If Action Subsystem2/1(prin)
  Merge/1 -> Mux/2
  Mux/1 -> Data Type Conversion3/1
  If Action Subsystem2/1(prout) -> Merge/1
  If/2 -> If Action Subsystem2/Action
  Logical Operator/1 -> If/1
  If/1 -> If Action Subsystem/Action
  Selector1/1 -> Product/2, Data Type Conversion1/1
  Data Type Conversion2/1 -> Math Function/1
  Data Type Conversion3/1 -> Memory/1, orient_estimaout/1
  Selector5/1 -> Sum/1, Wbe/1(rpy)
  Data Type Conversion1/1 -> dorient_estimaout/1
  Selector4/1 -> Mux/1

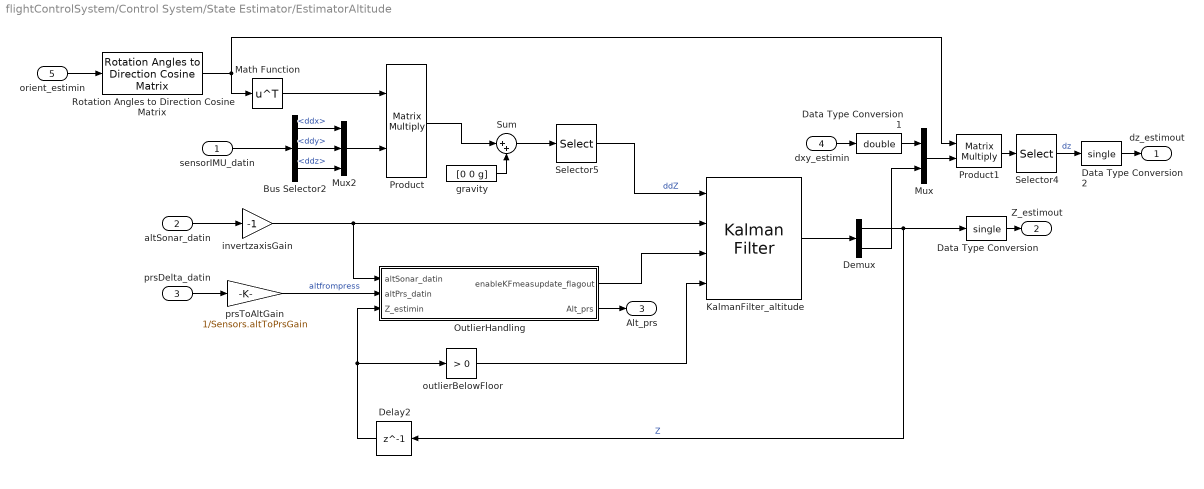
== system flightControlSystem/Control System/State Estimator/EstimatorAltitude ==
  sensorIMU_datin : Inport
  altSonar_datin : Inport  Port=2
  prsDelta_datin : Inport  Port=3
  dxy_estimin : Inport  Port=4
  orient_estimin : Inport  Port=5
  Bus Selector2 : BusSelector  OutputSignals=ddx,ddy,ddz
  Data Type Conversion : DataTypeConversion  OutDataTypeStr=single  SaturateOnIntegerOverflow=on
  Data Type Conversion1 : DataTypeConversion  OutDataTypeStr=double  SaturateOnIntegerOverflow=on
  Data Type Conversion2 : DataTypeConversion  OutDataTypeStr=single  SaturateOnIntegerOverflow=on
  Delay2 : Delay  DelayLength=1  InitialCondition=0
  Demux : Demux  Outputs=2
  KalmanFilter_altitude : ctrlSharedLib/Kalman Filter  TimeDomain=Discrete-Time  UseCurrentEstimator=on  ModelSource=Individual A, B, C, D matrices  ModelSourceVariable=sys  A=[1 Ts; 0 1]  B=[0;Ts]  C=[1 0]  D=[0]  NumberOfStates=2  NumberOfInputs=2  NumberOfOutputs=2  InitialEstimateSource=Dialog  X0=[init.posNED(3) 0]  P0=10  UseK=off  UseGH=on  NumberOfProcessNoiseInputs=2  G=Estimator.alt.kf.G  TimeInvariantG=on  H=Estimator.alt.kf.H  TimeInvariantH=on  Q=Estimator.alt.kf.Q  TimeInvariantQ=on  R=Estimator.alt.kf.R  TimeInvariantR=on  N=Estimator.alt.kf.N  TimeInvariantN=on  AddInputPort=on  AddEnablePort=on  ExternalReset=Level hold  OutputEstimatedY=off  OutputP=off  Ts=-1
      settings: SourceProductBaseCode=CT
  Math Function : Math  Operator=transpose  SaturateOnIntegerOverflow=on
  Mux : Mux  Inputs=2
  Mux2 : Mux  Inputs=3
  OutlierHandling : Subsystem
  Product : Product  Multiplication=Matrix(*)
  Product1 : Product  Multiplication=Matrix(*)
  Rotation Angles to Direction Cosine Matrix : sharedtransform/Rotation Angles to Direction Cosine Matrix  rotationOrder=ZYX  aMode=aMode
      settings: SourceProductBaseCode=AE
  Selector4 : Selector  InputPortWidth=3  IndexOptions=Index vector (dialog)  Indices=[3]  OutputSizes=1
  Selector5 : Selector  InputPortWidth=3  IndexOptions=Index vector (dialog)  Indices=[3]  OutputSizes=1
  Sum : Sum  Inputs=|++
  gravity : Constant  Value=[0 0 g]
  invertzaxisGain : Gain  Gain=-1  ParamDataTypeStr=single  OutDataTypeStr=double
  outlierBelowFloor : simulink/Logic and Bit Operations/Compare To Constant  relop=>  const=0  OutDataTypeStr=boolean
  prsToAltGain : Gain  Gain=1/Sensors.altToPrsGain
  dz_estimout : Outport
  Z_estimout : Outport  Port=2
  Alt_prs : Outport  Port=3
  wires:
  Mux2/1 -> Product/2
  sensorIMU_datin/1 -> Bus Selector2/1
  Bus Selector2/3 -> Mux2/3  "<ddz>"
  Bus Selector2/2 -> Mux2/2  "<ddy>"
  Bus Selector2/1 -> Mux2/1  "<ddx>"
  Product1/1 -> Selector4/1
  dxy_estimin/1 -> Data Type Conversion1/1
  Delay2/1 -> OutlierHandling/3(Z_estimin), outlierBelowFloor/1
  prsToAltGain/1 -> OutlierHandling/2(altPrs_datin)  "altfrompress"
  prsDelta_datin/1 -> prsToAltGain/1
  outlierBelowFloor/1 -> KalmanFilter_altitude/4
  Demux/2 -> Mux/2
  Selector4/1 -> Data Type Conversion2/1  "dz"
  Demux/1 -> Data Type Conversion/1, Delay2/1  "Z"
  Selector5/1 -> KalmanFilter_altitude/1  "ddZ"
  Mux/1 -> Product1/2
  KalmanFilter_altitude/1 -> Demux/1
  Sum/1 -> Selector5/1
  gravity/1 -> Sum/2
  Product/1 -> Sum/1
  altSonar_datin/1 -> invertzaxisGain/1
  orient_estimin/1 -> Rotation Angles to Direction Cosine Matrix/1
  Data Type Conversion/1 -> Z_estimout/1
  Data Type Conversion1/1 -> Mux/1
  Math Function/1 -> Product/1
  invertzaxisGain/1 -> KalmanFilter_altitude/2, OutlierHandling/1(altSonar_datin)
  Data Type Conversion2/1 -> dz_estimout/1
  OutlierHandling/1(enableKFmeasupdate_flagout) -> KalmanFilter_altitude/3
  Rotation Angles to Direction Cosine Matrix/1 -> Math Function/1, Product1/1
  OutlierHandling/2(Alt_prs) -> Alt_prs/1

== system flightControlSystem/Control System/State Estimator/EstimatorXYPosition ==
  opticalFlow_datin : Inport
  controlModePosVSOrient_flagin : Inport  Port=2
  sensorIMU_datin : Inport  Port=3
  Z_estimin : Inport  Port=4
  dz_estimin : Inport  Port=5
  orient_estimin : Inport  Port=6
  EstimatorVelocity : Subsystem
  EstimatorXYPosition : Subsystem
  XY_estimout : Outport
  dxy_estimout : Outport  Port=2
  wires:
  EstimatorXYPosition/1(XY_estimout) -> XY_estimout/1
  dz_estimin/1 -> EstimatorXYPosition/4(dz_estimin)
  controlModePosVSOrient_flagin/1 -> EstimatorXYPosition/3(controlModePosVSOrient_flagin)
  Z_estimin/1 -> EstimatorVelocity/2(Z_estimin)
  sensorIMU_datin/1 -> EstimatorVelocity/3(sensorIMU_datin)
  opticalFlow_datin/1 -> EstimatorVelocity/1(opticalFlow_datin)
  EstimatorVelocity/1(dxy_estimout) -> dxy_estimout/1, EstimatorXYPosition/1(dxy_estimin)
  orient_estimin/1 -> EstimatorVelocity/4(orient_estimin), EstimatorXYPosition/2(orient_estimin)

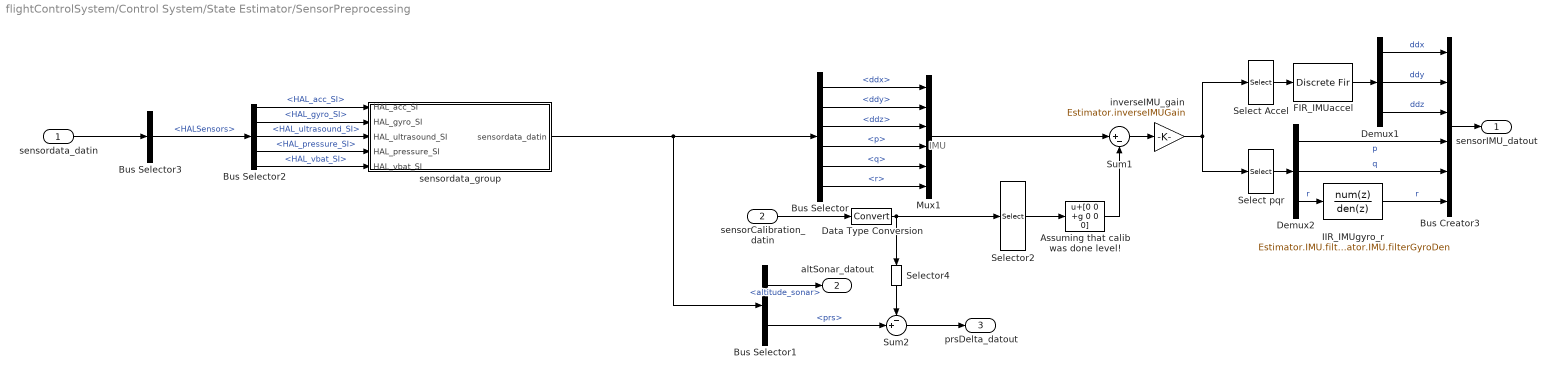
== system flightControlSystem/Control System/State Estimator/SensorPreprocessing ==
  note: IMU
  sensordata_datin : Inport
  sensorCalibration_datin : Inport  Port=2
  Assuming that calib was done level! : Bias  Bias=[0 0 +g 0 0 0]
  Bus Creator3 : BusCreator  Inputs=6
  Bus Selector : BusSelector  OutputSignals=ddx,ddy,ddz,p,q,r
  Bus Selector1 : BusSelector  OutputSignals=altitude_sonar,prs
  Bus Selector2 : BusSelector  OutputSignals=HAL_acc_SI,HAL_gyro_SI,HAL_ultrasound_SI,HAL_pressure_SI,HAL_vbat_SI
  Bus Selector3 : BusSelector  OutputSignals=HALSensors
  Data Type Conversion : DataTypeConversion
  Demux1 : Demux  Outputs=3
  Demux2 : Demux  Outputs=3
  FIR_IMUaccel : DiscreteFir  Coefficients=Estimator.IMU.filterAccel.Coefficients
  IIR_IMUgyro_r : DiscreteFilter  Numerator=Estimator.IMU.filterGyroNum  Denominator=Estimator.IMU.filterGyroDen
  Mux1 : Mux  Inputs=6
  Select Accel : Selector  InputPortWidth=6  IndexOptions=Index vector (dialog)  Indices=[1 2 3]  OutputSizes=1
  Select pqr : Selector  InputPortWidth=6  IndexOptions=Index vector (dialog)  Indices=[4 5 6]  OutputSizes=1
  Selector2 : Selector  InputPortWidth=8  IndexOptions=Index vector (dialog)  Indices=[1:6]  OutputSizes=1
  Selector4 : Selector  InputPortWidth=8  IndexOptions=Index vector (dialog)  Indices=[7]  OutputSizes=1
  Sum1 : Sum  Inputs=|+-
  Sum2 : Sum  Inputs=-+|
  inverseIMU_gain : Gain  Gain=Estimator.inverseIMUGain  ParamDataTypeStr=single  OutDataTypeStr=single
  sensordata_group : Subsystem
  sensorIMU_datout : Outport
  altSonar_datout : Outport  Port=2
  prsDelta_datout : Outport  Port=3
  wires:
  Select pqr/1 -> Demux2/1
  Assuming that calib was done level!/1 -> Sum1/2
  Mux1/1 -> Sum1/1
  Sum2/1 -> prsDelta_datout/1
  Bus Selector1/2 -> Sum2/2  "<prs>"
  Selector4/1 -> Sum2/1
  Bus Selector1/1 -> altSonar_datout/1  "<altitude_sonar>"
  Bus Selector/6 -> Mux1/6  "<r>"
  Bus Selector/5 -> Mux1/5  "<q>"
  Bus Selector/4 -> Mux1/4  "<p>"
  Bus Selector/3 -> Mux1/3  "<ddz>"
  Bus Selector/2 -> Mux1/2  "<ddy>"
  Bus Selector/1 -> Mux1/1  "<ddx>"
  sensorCalibration_datin/1 -> Data Type Conversion/1
  IIR_IMUgyro_r/1 -> Bus Creator3/6  "r"
  Demux2/3 -> IIR_IMUgyro_r/1  "r"
  FIR_IMUaccel/1 -> Demux1/1
  Select Accel/1 -> FIR_IMUaccel/1
  inverseIMU_gain/1 -> Select Accel/1, Select pqr/1
  Demux2/2 -> Bus Creator3/5  "q"
  Demux2/1 -> Bus Creator3/4  "p"
  Selector2/1 -> Assuming that calib was done level!/1
  Sum1/1 -> inverseIMU_gain/1
  Demux1/3 -> Bus Creator3/3  "ddz"
  Demux1/2 -> Bus Creator3/2  "ddy"
  Demux1/1 -> Bus Creator3/1  "ddx"
  Bus Creator3/1 -> sensorIMU_datout/1
  Data Type Conversion/1 -> Selector2/1, Selector4/1
  Bus Selector2/2 -> sensordata_group/2(HAL_gyro_SI)  "<HAL_gyro_SI>"
  Bus Selector2/4 -> sensordata_group/4(HAL_pressure_SI)  "<HAL_pressure_SI>"
  Bus Selector2/5 -> sensordata_group/5(HAL_vbat_SI)  "<HAL_vbat_SI>"
  Bus Selector2/3 -> sensordata_group/3(HAL_ultrasound_SI)  "<HAL_ultrasound_SI>"
  Bus Selector3/1 -> Bus Selector2/1  "<HALSensors>"
  sensordata_group/1(sensordata_datin) -> Bus Selector1/1, Bus Selector/1
  sensordata_datin/1 -> Bus Selector3/1
  Bus Selector2/1 -> sensordata_group/1(HAL_acc_SI)  "<HAL_acc_SI>"

== system flightControlSystem/Control System/State Estimator/Complementary Filter/If Action Subsystem ==
  rpy : Inport
  accel : Inport  Port=2
  Action Port : ActionPort  ActionPortLabel=if(u1 > 0)
  Demux : Demux  Outputs=3
  Demux1 : Demux  Outputs=3
  Divide : Product  Inputs=*/
  Gain : Gain  Gain=1-Estimator.gyroAngleUpdateAccWeight
  Gain1 : Gain  Gain=Estimator.gyroAngleUpdateAccWeight
  Gain2 : Gain  Gain=1/g
  Gain3 : Gain  Gain=Estimator.gyroAngleUpdateAccWeight
  Gain4 : Gain  Gain=1-Estimator.gyroAngleUpdateAccWeight
  Mux : Mux  Inputs=2
  Sum : Sum  Inputs=|++
  Sum1 : Sum  Inputs=|++
  Terminator1 : Terminator
  Trigonometric Function : Trigonometry  Operator=atan
  Trigonometric Function1 : Trigonometry  Operator=asin
  pitch,roll : Outport
  wires:
  accel/1 -> Demux/1
  Demux/2 -> Divide/1
  Demux/3 -> Divide/2
  Divide/1 -> Trigonometric Function/1
  Gain/1 -> Sum/1
  Trigonometric Function/1 -> Gain1/1
  Mux/1 -> pitch,roll/1
  Gain2/1 -> Trigonometric Function1/1
  Trigonometric Function1/1 -> Gain3/1
  Gain4/1 -> Sum1/1
  Gain3/1 -> Sum1/2
  Sum1/1 -> Mux/1
  Sum/1 -> Mux/2
  rpy/1 -> Demux1/1
  Demux1/1 -> Gain/1
  Demux1/2 -> Gain4/1
  Demux/1 -> Gain2/1
  Demux1/3 -> Terminator1/1
  Gain1/1 -> Sum/2

== system flightControlSystem/Control System/State Estimator/Complementary Filter/If Action Subsystem2 ==
  prin : Inport
  Action Port : ActionPort  ActionPortLabel=else
  prout : Outport
  wires:
  prin/1 -> prout/1

== system flightControlSystem/Control System/State Estimator/Complementary Filter/Wbe ==
  rpy : Inport  OutDataTypeStr=single
  Constant : Constant  Value=single(0)
  Create 3x3 Matrix : sharedutil/Create 3x3 Matrix  aMode=aMode
  Divide : Product  Inputs=*/
  Gain : Gain  Gain=-1
  Product{1..4} (4 alike) : Product
  Selector : Selector  InputPortWidth=3  IndexOptions=Index vector (dialog)  Indices=[1]  OutputSizes=1
  Selector1 : Selector  InputPortWidth=3  IndexOptions=Index vector (dialog)  Indices=[1]  OutputSizes=1
  Selector2 : Selector  InputPortWidth=3  IndexOptions=Index vector (dialog)  Indices=[2]  OutputSizes=1
  Selector3 : Selector  InputPortWidth=3  IndexOptions=Index vector (dialog)  Indices=[2]  OutputSizes=1
  Trigonometric Function : Trigonometry  Operator=sincos
  Wbe : Outport
  wires:
  Create 3x3 Matrix/1 -> Divide/1
  Product3/1 -> Create 3x3 Matrix/8
  Trigonometric Function/2 -> Selector1/1, Selector2/1
  Selector3/1 -> Product4/2, Product3/2
  Selector1/1 -> Product4/1, Product1/1, Create 3x3 Matrix/3
  Trigonometric Function/1 -> Selector3/1, Selector/1
  Product1/1 -> Create 3x3 Matrix/5
  Product2/1 -> Create 3x3 Matrix/6
  Selector2/1 -> Divide/2, Create 3x3 Matrix/7, Product2/1, Product1/2
  Gain/1 -> Product2/2
  Product4/1 -> Create 3x3 Matrix/9
  Constant/1 -> Create 3x3 Matrix/4, Create 3x3 Matrix/1
  Divide/1 -> Wbe/1
  rpy/1 -> Trigonometric Function/1
  Selector/1 -> Product3/1, Gain/1, Create 3x3 Matrix/2

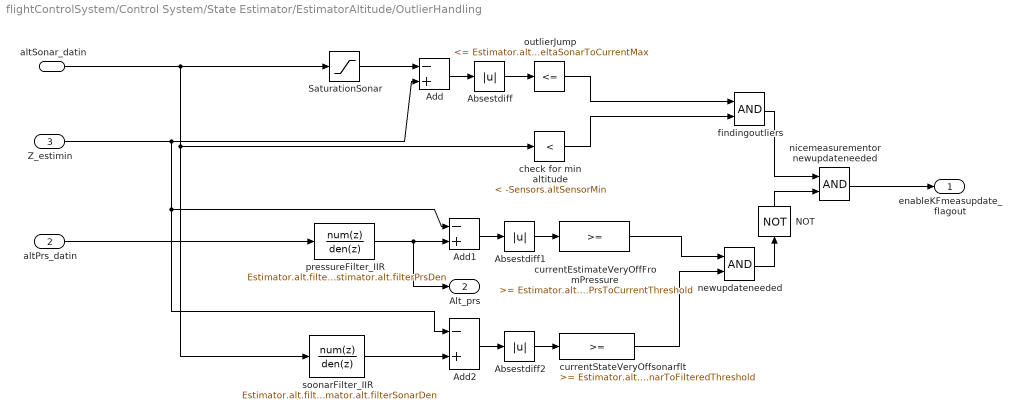
== system flightControlSystem/Control System/State Estimator/EstimatorAltitude/OutlierHandling ==
  altSonar_datin : Inport
  altPrs_datin : Inport  Port=2
  Z_estimin : Inport  Port=3
  Absestdiff : Abs
  Absestdiff1 : Abs
  Absestdiff2 : Abs
  Add : Sum  Inputs=-+
  Add1 : Sum  Inputs=-+
  Add2 : Sum  Inputs=-+
  NOT : Logic  Operator=NOT  IconShape=distinctive  AllPortsSameDT=off  OutDataTypeStr=boolean
  SaturationSonar : Saturate  UpperLimit=-Sensors.altSensorMin  LowerLimit=-inf
  check for min altitude : simulink/Logic and Bit Operations/Compare To Constant  relop=<  const=-Sensors.altSensorMin  OutDataTypeStr=boolean
  currentEstimateVeryOffFromPressure : simulink/Logic and Bit Operations/Compare To Constant  relop=>=  const=Estimator.alt.deltaPrsToCurrentThreshold  OutDataTypeStr=boolean
  currentStateVeryOffsonarflt : simulink/Logic and Bit Operations/Compare To Constant  relop=>=  const=Estimator.alt.deltaSonarToFilteredThreshold  OutDataTypeStr=boolean
  findingoutliers : Logic  AllPortsSameDT=off  OutDataTypeStr=boolean
  newupdateneeded : Logic  AllPortsSameDT=off  OutDataTypeStr=boolean
  nicemeasurementor newupdateneeded : Logic  AllPortsSameDT=off  OutDataTypeStr=boolean
  outlierJump : simulink/Logic and Bit Operations/Compare To Constant  relop=<=  const=Estimator.alt.deltaSonarToCurrentMax  OutDataTypeStr=boolean
  pressureFilter_IIR : DiscreteFilter  Numerator=Estimator.alt.filterPrsNum  Denominator=Estimator.alt.filterPrsDen
  soonarFilter_IIR : DiscreteFilter  Numerator=Estimator.alt.filterSonarNum  Denominator=Estimator.alt.filterSonarDen
  enableKFmeasupdate_flagout : Outport
  Alt_prs : Outport  Port=2
  wires:
  Add1/1 -> Absestdiff1/1
  nicemeasurementor newupdateneeded/1 -> enableKFmeasupdate_flagout/1
  findingoutliers/1 -> nicemeasurementor newupdateneeded/1
  check for min altitude/1 -> findingoutliers/2
  outlierJump/1 -> findingoutliers/1
  SaturationSonar/1 -> Add/1
  Absestdiff/1 -> outlierJump/1
  Add/1 -> Absestdiff/1
  newupdateneeded/1 -> NOT/1
  Absestdiff2/1 -> currentStateVeryOffsonarflt/1
  altSonar_datin/1 -> SaturationSonar/1, soonarFilter_IIR/1, check for min altitude/1
  currentEstimateVeryOffFromPressure/1 -> newupdateneeded/1
  Z_estimin/1 -> Add1/1, Add2/1, Add/2
  Add2/1 -> Absestdiff2/1
  currentStateVeryOffsonarflt/1 -> newupdateneeded/2
  pressureFilter_IIR/1 -> Alt_prs/1, Add1/2
  altPrs_datin/1 -> pressureFilter_IIR/1
  soonarFilter_IIR/1 -> Add2/2
  Absestdiff1/1 -> currentEstimateVeryOffFromPressure/1
  NOT/1 -> nicemeasurementor newupdateneeded/2

== system flightControlSystem/Control System/State Estimator/EstimatorXYPosition/EstimatorVelocity ==
  opticalFlow_datin : Inport
  Z_estimin : Inport  Port=2  SampleTime=Ts
  sensorIMU_datin : Inport  Port=3
  orient_estimin : Inport  Port=4
  " " : Product  Inputs=**
  AccelerationHandling : Subsystem
  Compare To Constant : simulink/Logic and Bit Operations/Compare To Constant  relop=<  const=200*4  OutDataTypeStr=boolean
  Counter Free-Running : simulink/Sources/Counter Free-Running  NumBits=32  tsamp=-1
  DataHandling : Subsystem
  Delay : Delay  DelayLength=1  InitialCondition=0
  Gain : Gain  Gain=-1
  KalmanFilter_dxdy : ctrlSharedLib/Kalman Filter  TimeDomain=Discrete-Time  UseCurrentEstimator=on  ModelSource=Individual A, B, C, D matrices  ModelSourceVariable=ss(0.95,1,1,0,1)  A=eye(2)  B=Ts*eye(2)  C=eye(2)  D=0  NumberOfStates=1  NumberOfInputs=1  NumberOfOutputs=1  InitialEstimateSource=Dialog  X0=0  P0=10  UseK=off  UseGH=on  NumberOfProcessNoiseInputs=1  G=Estimator.pos.kfVelo.G  TimeInvariantG=on  H=Estimator.pos.kfVelo.H  TimeInvariantH=on  Q=Estimator.pos.kfVelo.Q  TimeInvariantQ=on  R=Estimator.pos.kfVelo.R  TimeInvariantR=on  N=Estimator.pos.kfVelo.N  TimeInvariantN=on  AddInputPort=on  AddEnablePort=on  OutputEstimatedY=off  OutputP=off  Ts=-1
      settings: SourceProductBaseCode=CT
  Select dxy : Selector  InputPortWidth=3  IndexOptions=Index vector (dialog)  Indices=[1 2]  OutputSizes=1
  Switch : Switch  Criteria=u2 > Threshold
  Z_estimin1 : InportShadow  Port=2  SampleTime=Ts
  opticalFlowErrorCorrect : Gain  Gain=1.15
  dxy_estimout : Outport
  wires:
  Delay/1 -> DataHandling/5(dxyOF_datin)
  Z_estimin/1 -> DataHandling/1(Z_estimin), AccelerationHandling/4(Z_estimin)
  KalmanFilter_dxdy/1 -> dxy_estimout/1, Delay/1
  sensorIMU_datin/1 -> AccelerationHandling/2(sensorIMU_datin), DataHandling/3(sensorIMU_datin)
  orient_estimin/1 -> AccelerationHandling/3(orient_estimin), DataHandling/2(orient_estimin)
  Select dxy/1 -> KalmanFilter_dxdy/2, AccelerationHandling/1(dxy_estimin), DataHandling/4(dxy_estimin)
  AccelerationHandling/1(acceleration_world) -> KalmanFilter_dxdy/1
  DataHandling/1(enable_flag) -> KalmanFilter_dxdy/3
  Switch/1 -> Select dxy/1
  " "/1 -> opticalFlowErrorCorrect/1
  Gain/1 -> " "/2
  opticalFlowErrorCorrect/1 -> Switch/3
  Compare To Constant/1 -> Switch/2
  opticalFlow_datin/1 -> " "/1, Switch/1
  Z_estimin1/1 -> Gain/1
  Counter Free-Running/1 -> Compare To Constant/1

== system flightControlSystem/Control System/State Estimator/EstimatorXYPosition/EstimatorXYPosition ==
  note: Switching from orientationControl to Position
      | control reset the current world position estimate
      | (happens when using no markers)
  dxy_estimin : Inport
  orient_estimin : Inport  Port=2  SampleTime=Ts
  controlModePosVSOrient_flagin : Inport  Port=3
  dz_estimin : Inport  Port=4
  Math Function : Math  Operator=transpose  SaturateOnIntegerOverflow=on
  Mux2 : Mux  Inputs=2
  Product : Product  Multiplication=Matrix(*)
  Rotation Angles to Direction Cosine Matrix : sharedtransform/Rotation Angles to Direction Cosine Matrix  rotationOrder=ZYX  aMode=aMode
      settings: SourceProductBaseCode=AE
  SelectdXY : Selector  InputPortWidth=3  IndexOptions=Index vector (dialog)  Indices=[1 2]  OutputSizes=1
  SimplyIntegrateVelocity : DiscreteIntegrator  ExternalReset=rising  SampleTime=Ts  ICPrevOutput=DiscIntNeverNeededParam  ICPrevScaledInput=DiscIntNeverNeededParam
  XY_estimout : Outport
  wires:
  controlModePosVSOrient_flagin/1 -> SimplyIntegrateVelocity/2
  Product/1 -> SelectdXY/1
  Mux2/1 -> Product/2
  dz_estimin/1 -> Mux2/2
  SimplyIntegrateVelocity/1 -> XY_estimout/1
  dxy_estimin/1 -> Mux2/1
  orient_estimin/1 -> Rotation Angles to Direction Cosine Matrix/1
  Rotation Angles to Direction Cosine Matrix/1 -> Math Function/1
  SelectdXY/1 -> SimplyIntegrateVelocity/1
  Math Function/1 -> Product/1
